simulink model "sf_abstemporal_basic"  (Simulink 7.6)
settings: Solver=FixedStepDiscrete  StartTime=0.0  StopTime=10.0  FixedStep=0.1  RelTol=1e-3
settings Model: Creator=The MathWorks Inc.
settings DebuggingCC: StrictBusMsg=Warning
settings SFSimCC: SimParseCustomCode=off

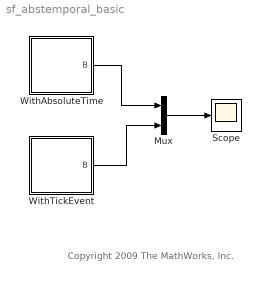
== system sf_abstemporal_basic ==
  note: Copyright 2009 The MathWorks, Inc.
  Mux : Mux  Inputs=2
  Scope : Scope
      settings: YMin=0  YMax=1
  WithAbsoluteTime : Stateflow chart  TreatAsAtomicUnit=on
  WithTickEvent : Stateflow chart  TreatAsAtomicUnit=on
  wires:
  WithTickEvent/1(B) -> Mux/2
  Mux/1 -> Scope/1
  WithAbsoluteTime/1(B) -> Mux/1

== stateflow chart WithAbsoluteTime ==
  state A
  state B
  (default) -> A
  A -> B : after(3,sec)
  data: B output boolean

== stateflow chart WithTickEvent ==
  state A
  state B
  (default) -> A
  A -> B : after(30,tick)
  data: B output boolean
